simulink model "TP_ABS_GUIVARCH"  (R2022b)
settings: Solver=ode45  StartTime=0.0  StopTime=10  RelTol=1e-3
InitFcn:
  | Cte_TP_ABS_CHERIF
values from neighbouring files (symbols this model uses):
  f = 0.8    [Cte_TP_ABS_CHERIF.m]
  g = 9.81    [Cte_TP_ABS_CHERIF.m]    (also in Cte_Traction.m)
  J = 0.5    [Cte_TP_ABS_CHERIF.m]    (also in Cte_Traction.m)
  Kd = 0    [Cte_TP_ABS_CHERIF.m]
  Ki = 10    [Cte_TP_ABS_CHERIF.m]
  Kp = 100    [Cte_TP_ABS_CHERIF.m]
  m = 1000    [Cte_TP_ABS_CHERIF.m]    (also in Cte_Traction.m = 1500)
  rRoue = 0.3    [Cte_TP_ABS_CHERIF.m]
  Ts = 0,0001    [Cte_TP_ABS_CHERIF.m]
  v0 = 27.77    [Cte_TP_ABS_CHERIF.m]
undefined symbols (not defined in the file or in its folder): DiscIntNeverNeededParam
libraries: simulink x1
settings Model: Creator=enzoc  LastModifiedBy=enzoc
settings OptimizationCC: ReuseModelBlockBuffer=on
settings DebuggingCC: AlgebraicLoopMsg=none
settings RTWCC: GPUComputeCapability=5.0

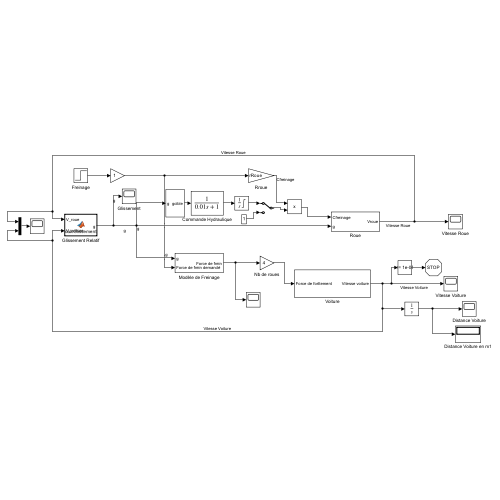
[thumbnail: Simulink's stored preview of the top-level diagram]
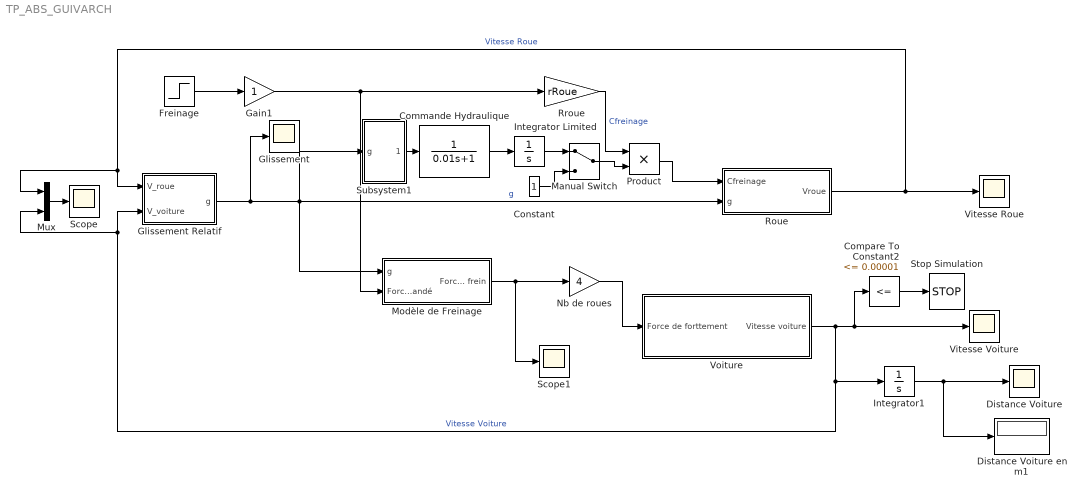
== system TP_ABS_GUIVARCH ==
  Commande Hydraulique : TransferFcn  Denominator=[0.01 1]
  Compare To Constant2 : simulink/Logic and Bit Operations/Compare To Constant  relop=<=  const=0.00001  OutDataTypeStr=boolean
  Constant : Constant
  Distance Voiture : Scope
  Distance Voiture en m1 : Display
  Freinage : Step  Time=0  After=6000  SampleTime=0
  Gain1 : Gain
  Glissement : Scope
  Glissement Relatif : MATLAB Function  TreatAsAtomicUnit=on
  Integrator Limited : Integrator  LimitOutput=on  UpperSaturationLimit=1000  LowerSaturationLimit=0
  Integrator1 : Integrator
  Manual Switch : ManualSwitch
  Modèle de Freinage : Subsystem
  Mux : Mux  Inputs=2
  Nb de roues : Gain  Gain=4
  Product : Product
  Roue : Subsystem
  Rroue : Gain  Gain=rRoue
  Scope : Scope
  Scope1 : Scope
  Stop Simulation : Stop
  Subsystem1 : Subsystem
  Vitesse Roue : Scope
  Vitesse Voiture : Scope
  Voiture : Subsystem
  wires:
  Glissement Relatif/1(g) -> Glissement/1, Subsystem1/1(g), Roue/2(g), Modèle de Freinage/1(g)  "g"
  Nb de roues/1 -> Voiture/1(Force de forttement)
  Voiture/1(Vitesse voiture) -> Integrator1/1, Mux/2, Glissement Relatif/2(V_voiture), Compare To Constant2/1, Vitesse Voiture/1  "Vitesse Voiture"
  Modèle de Freinage/1(Force de frein) -> Nb de roues/1, Scope1/1
  Freinage/1 -> Gain1/1
  Roue/1(Vroue) -> Vitesse Roue/1, Mux/1, Glissement Relatif/1(V_roue)  "Vitesse Roue"
  Integrator1/1 -> Distance Voiture/1, Distance Voiture en m1/1
  Mux/1 -> Scope/1
  Compare To Constant2/1 -> Stop Simulation/1
  Subsystem1/1(gcible) -> Commande Hydraulique/1
  Commande Hydraulique/1 -> Integrator Limited/1
  Gain1/1 -> Rroue/1, Modèle de Freinage/2(Force de frein demandé)
  Rroue/1 -> Product/1  "Cfreinage"
  Product/1 -> Roue/1(Cfreinage)
  Integrator Limited/1 -> Manual Switch/1
  Manual Switch/1 -> Product/2
  Constant/1 -> Manual Switch/2

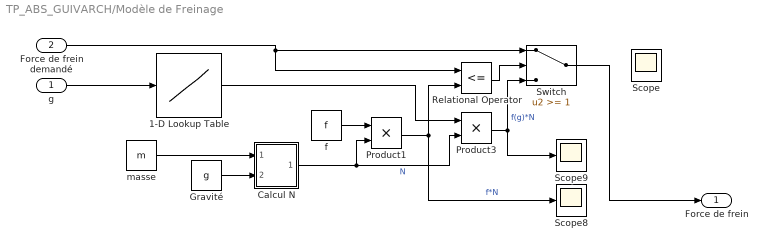
== system TP_ABS_GUIVARCH/Modèle de Freinage ==
  g : Inport
  Force de frein demandé : Inport  Port=2
  1-D Lookup Table : Lookup_n-D  NumberOfTableDimensions=1  BreakpointsForDimension1=[0;0.050000000000000003;0.10000000000000001;0.14999999999999999;0.20000000000000001;0.25;0.29999999999999999;0.34999999999999998;0.40000000000000002;0.45000000000000001;0.5;0.55000000000000004;0.59999999999999998;0.65000000000000002;0.69999999999999996;0.75;0.80000000000000004;0.84999999999999998;0.90000000000000002;0.94999999999999996;1]  Table=[0;0.59999999999999998;0.92000000000000004;0.93999999999999995;0.94999999999999996;0.93000000000000005;0.90000000000000002;0.84999999999999998;0.80000000000000004;0.75;0.69999999999999996;0.67000000000000004;0.66000000000000003;0.65000000000000002;0.64500000000000002;0.64000000000000001;0.63700000000000001;0.63500000000000001;0.63;0.625;0.62]  InternalRulePriority=Speed  RndMeth=Simplest
  Calcul N : Subsystem
  Gravité : Constant  Value=g
  Product1 : Product
  Product3 : Product
  Relational Operator : RelationalOperator  Operator=<=  OutDataTypeStr=boolean  RndMeth=Simplest  InputSameDT=off
  Scope : Scope
  Scope8 : Scope
  Scope9 : Scope
  Switch : Switch  Threshold=1  SaturateOnIntegerOverflow=off  InputSameDT=off
  f : Constant  Value=f
  masse : Constant  Value=m
  Force de frein : Outport
  wires:
  Force de frein demandé/1 -> Relational Operator/1, Switch/1
  masse/1 -> Calcul N/1(In1)
  Product3/1 -> Scope9/1, Switch/3  "f(g)*N"
  Product1/1 -> Scope8/1, Relational Operator/2  "f*N"
  Gravité/1 -> Calcul N/2(In2)
  Calcul N/1(Out1) -> Product3/2, Product1/2  "N"
  f/1 -> Product1/1
  Relational Operator/1 -> Switch/2
  g/1 -> 1-D Lookup Table/1
  1-D Lookup Table/1 -> Product3/1
  Switch/1 -> Force de frein/1

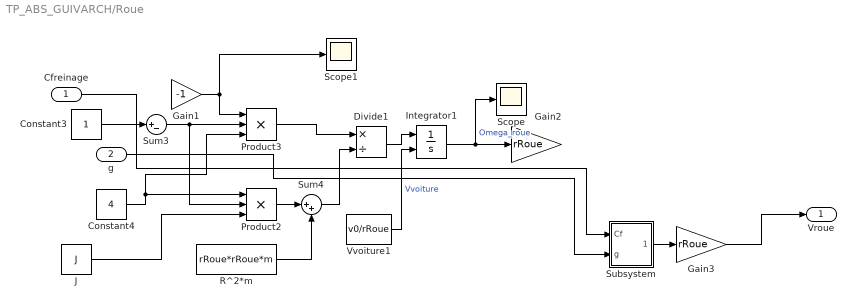
== system TP_ABS_GUIVARCH/Roue ==
  Cfreinage : Inport
  g : Inport  Port=2
  Constant3 : Constant
  Constant4 : Constant  Value=4
  Divide1 : Product  Inputs=*/
  Gain1 : Gain  Gain=-1
  Gain2 : Gain  Gain=rRoue
  Gain3 : Gain  Gain=rRoue
  Integrator1 : Integrator  InitialConditionSource=external  InitialCondition=27.77/0.3
  J : Constant  Value=J
  Product2 : Product  Inputs=3
  Product3 : Product  Inputs=3
  R^2*m : Constant  Value=rRoue*rRoue*m
  Scope : Scope
  Scope1 : Scope
  Subsystem : Subsystem
  Sum3 : Sum  Inputs=|+-
  Sum4 : Sum  Inputs=|++
  Vvoiture1 : Constant  Value=v0/rRoue
  Vroue : Outport
  wires:
  Divide1/1 -> Integrator1/1
  Gain1/1 -> Product3/1, Scope1/1
  Sum3/1 -> Product2/2, Product3/2
  Constant3/1 -> Sum3/1
  Vvoiture1/1 -> Integrator1/2  "Vvoiture"
  Product3/1 -> Divide1/1
  Product2/1 -> Sum4/1
  Sum4/1 -> Divide1/2
  Constant4/1 -> Product3/3, Product2/1
  J/1 -> Product2/3
  R^2*m/1 -> Sum4/2
  Integrator1/1 -> Scope/1, Gain2/1  "Omega_roue"
  Subsystem/1(Vroue) -> Gain3/1
  Cfreinage/1 -> Subsystem/1(Cf)
  g/1 -> Subsystem/2(g)
  Gain3/1 -> Vroue/1

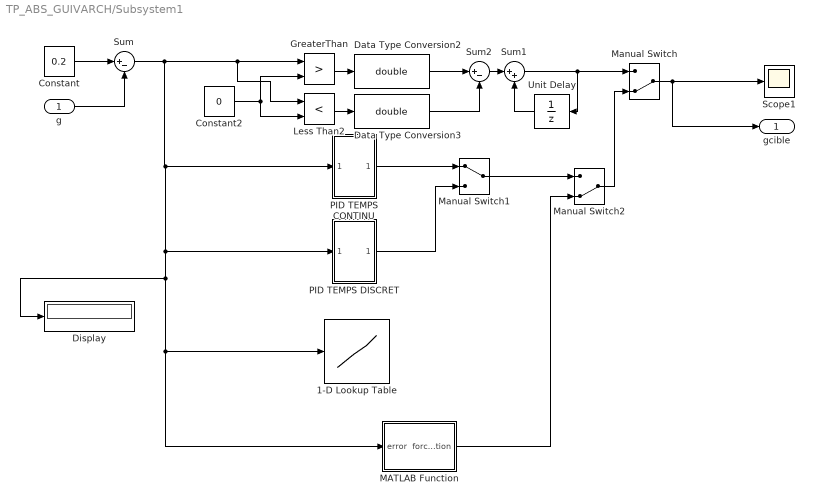
== system TP_ABS_GUIVARCH/Subsystem1 ==
  g : Inport
  1-D Lookup Table : Lookup_n-D  NumberOfTableDimensions=1  BreakpointsForDimension1=[-0.80000000000000004;-0.59999999999999998;-0.40000000000000002;-0.20000000000000001;0;0.10000000000000001;0.20000000000000001]  Table=[-800;-600;-400;-200;0;200;400]  InternalRulePriority=Speed  RndMeth=Simplest
  Constant : Constant  Value=0.2
  Constant2 : Constant  Value=0
  Data Type Conversion2 : DataTypeConversion  OutDataTypeStr=double  SaturateOnIntegerOverflow=off
  Data Type Conversion3 : DataTypeConversion  OutDataTypeStr=double  SaturateOnIntegerOverflow=off
  Display : Display
  GreaterThan : RelationalOperator  Operator=>  OutDataTypeStr=boolean  RndMeth=Simplest  InputSameDT=off
  Less Than2 : RelationalOperator  Operator=<  OutDataTypeStr=boolean  RndMeth=Simplest  InputSameDT=off
  MATLAB Function : MATLAB Function  TreatAsAtomicUnit=on
  Manual Switch : ManualSwitch  CurrentSetting=0
  Manual Switch1 : ManualSwitch
  Manual Switch2 : ManualSwitch  CurrentSetting=0
  PID TEMPS CONTINU : Subsystem
  PID TEMPS DISCRET : Subsystem
  Scope1 : Scope
  Sum : Sum  Inputs=|+-
  Sum1 : Sum  Inputs=|++
  Sum2 : Sum  Inputs=|+-
  Unit Delay : UnitDelay  SampleTime=0.0001  HasFrameUpgradeWarning=on
  gcible : Outport
  wires:
  Constant/1 -> Sum/1
  g/1 -> Sum/2
  GreaterThan/1 -> Data Type Conversion2/1
  Constant2/1 -> GreaterThan/2, Less Than2/2
  Data Type Conversion2/1 -> Sum2/1
  Less Than2/1 -> Data Type Conversion3/1
  Data Type Conversion3/1 -> Sum2/2
  Manual Switch/1 -> gcible/1, Scope1/1
  Sum/1 -> Display/1, MATLAB Function/1(error), 1-D Lookup Table/1, PID TEMPS DISCRET/1(In1), PID TEMPS CONTINU/1(In1), GreaterThan/1, Less Than2/1
  PID TEMPS CONTINU/1(Out1) -> Manual Switch1/1
  PID TEMPS DISCRET/1(Out1) -> Manual Switch1/2
  Sum2/1 -> Sum1/1
  Sum1/1 -> Unit Delay/1, Manual Switch/1
  Unit Delay/1 -> Sum1/2
  Manual Switch1/1 -> Manual Switch2/1
  Manual Switch2/1 -> Manual Switch/2
  MATLAB Function/1(force_correction) -> Manual Switch2/2

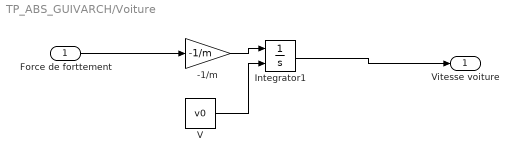
== system TP_ABS_GUIVARCH/Voiture ==
  Force de forttement : Inport
  -1/m : Gain  Gain=-1/m
  Integrator1 : Integrator  InitialConditionSource=external
  V : Constant  Value=v0
  Vitesse voiture : Outport
  wires:
  Force de forttement/1 -> -1/m/1
  -1/m/1 -> Integrator1/1
  Integrator1/1 -> Vitesse voiture/1
  V/1 -> Integrator1/2

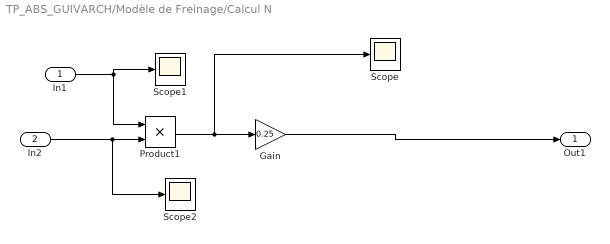
== system TP_ABS_GUIVARCH/Modèle de Freinage/Calcul N ==
  In1 : Inport
  In2 : Inport  Port=2
  Gain : Gain  Gain=0.25
  Product1 : Product
  Scope : Scope
  Scope1 : Scope
  Scope2 : Scope
  Out1 : Outport
  wires:
  Product1/1 -> Scope/1, Gain/1
  In1/1 -> Product1/1, Scope1/1
  In2/1 -> Scope2/1, Product1/2
  Gain/1 -> Out1/1

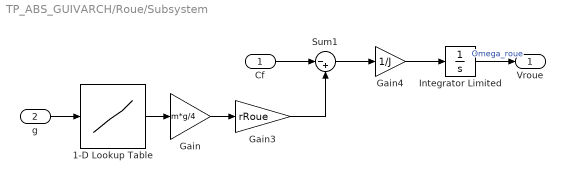
== system TP_ABS_GUIVARCH/Roue/Subsystem ==
  Cf : Inport
  g : Inport  Port=2
  1-D Lookup Table : Lookup_n-D  NumberOfTableDimensions=1  BreakpointsForDimension1=[0;0.050000000000000003;0.10000000000000001;0.14999999999999999;0.20000000000000001;0.25;0.29999999999999999;0.34999999999999998;0.40000000000000002;0.45000000000000001;0.5;0.55000000000000004;0.59999999999999998;0.65000000000000002;0.69999999999999996;0.75;0.80000000000000004;0.84999999999999998;0.90000000000000002;0.94999999999999996;1]  Table=[0;0.59999999999999998;0.92000000000000004;0.93999999999999995;0.94999999999999996;0.93000000000000005;0.90000000000000002;0.84999999999999998;0.80000000000000004;0.75;0.69999999999999996;0.67000000000000004;0.66000000000000003;0.65000000000000002;0.64500000000000002;0.64000000000000001;0.63700000000000001;0.63500000000000001;0.63;0.625;0.62]  InternalRulePriority=Speed  RndMeth=Simplest
  Gain : Gain  Gain=m*g/4
  Gain3 : Gain  Gain=rRoue
  Gain4 : Gain  Gain=1/J
  Integrator Limited : Integrator  InitialCondition=v0/rRoue  LimitOutput=on  UpperSaturationLimit=1000  LowerSaturationLimit=0
  Sum1 : Sum  Inputs=|-+
  Vroue : Outport
  wires:
  Integrator Limited/1 -> Vroue/1  "Omega_roue"
  Gain4/1 -> Integrator Limited/1
  Gain/1 -> Gain3/1
  Cf/1 -> Sum1/1
  Gain3/1 -> Sum1/2
  Sum1/1 -> Gain4/1
  g/1 -> 1-D Lookup Table/1
  1-D Lookup Table/1 -> Gain/1

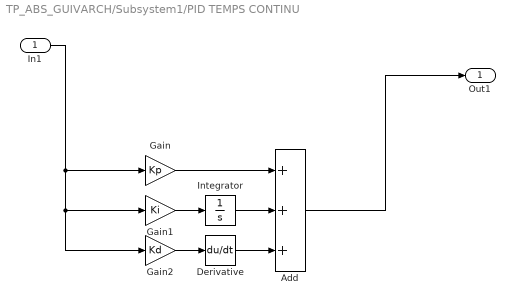
== system TP_ABS_GUIVARCH/Subsystem1/PID TEMPS CONTINU ==
  In1 : Inport
  Add : Sum  Inputs=+++
  Derivative : Derivative
  Gain : Gain  Gain=Kp
  Gain1 : Gain  Gain=Ki
  Gain2 : Gain  Gain=Kd
  Integrator : Integrator
  Out1 : Outport
  wires:
  Derivative/1 -> Add/3
  Add/1 -> Out1/1
  In1/1 -> Gain2/1, Gain1/1, Gain/1
  Gain/1 -> Add/1
  Gain2/1 -> Derivative/1
  Integrator/1 -> Add/2
  Gain1/1 -> Integrator/1

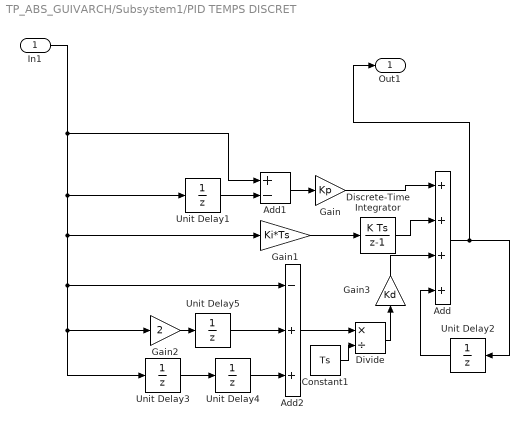
== system TP_ABS_GUIVARCH/Subsystem1/PID TEMPS DISCRET ==
  In1 : Inport
  Add : Sum  Inputs=++++
  Add1 : Sum  Inputs=+-
  Add2 : Sum  Inputs=-++
  Constant1 : Constant  Value=Ts
  Discrete-Time Integrator : DiscreteIntegrator  SampleTime=-1  ICPrevOutput=DiscIntNeverNeededParam  ICPrevScaledInput=DiscIntNeverNeededParam
  Divide : Product  Inputs=*/
  Gain : Gain  Gain=Kp
  Gain1 : Gain  Gain=Ki*Ts
  Gain2 : Gain  Gain=2
  Gain3 : Gain  Gain=Kd
  Unit Delay{1..5} (5 alike) : UnitDelay  SampleTime=0.0001  HasFrameUpgradeWarning=on
  Out1 : Outport
  wires:
  In1/1 -> Unit Delay3/1, Gain2/1, Add2/1, Gain1/1, Unit Delay1/1, Add1/1
  Gain2/1 -> Unit Delay5/1
  Add/1 -> Out1/1, Unit Delay2/1
  Constant1/1 -> Divide/2
  Divide/1 -> Gain3/1
  Unit Delay4/1 -> Add2/3
  Unit Delay5/1 -> Add2/2
  Gain3/1 -> Add/3
  Add2/1 -> Divide/1
  Unit Delay2/1 -> Add/4
  Unit Delay3/1 -> Unit Delay4/1
  Gain1/1 -> Discrete-Time Integrator/1
  Unit Delay1/1 -> Add1/2
  Gain/1 -> Add/1
  Discrete-Time Integrator/1 -> Add/2
  Add1/1 -> Gain/1

== matlab function TP_ABS_GUIVARCH/Glissement Relatif ==
  data: V_roue input; V_voiture input; g output
function g = calcGlissement(V_roue, V_voiture)
    g = 1 - (V_roue / V_voiture);

end

== matlab function TP_ABS_GUIVARCH/Subsystem1/MATLAB Function ==
  settings: updateMethod=DISCRETE
  data: error input; force_correction output
function force_correction = ABS_Control(error)
    % Définir les limites de la force de freinage
    max_force = 800;
    min_force = -800;

    % Initialiser la force de correction
    persistent current_force
    if isempty(current_force)
        current_force = 0;  % Valeur initiale de la force de freinage
    end

    % Ajustement de la force en fonction de l'erreur
    if error > 0.05
        % Si l'erreur est positive, augmenter la force de freinage
        current_force = current_force + 100;
    elseif error < -0.05
        % Si l'erreur est négative, diminuer la force de freinage
        current_force = current_force - 100;
    end

    % Appliquer les limites de saturation
    if current_force > max_force
        current_force = max_force;
    elseif current_force < min_force
        current_force = min_force;
    end

    % Sortie de la fonction
    force_correction = current_force;
end
